simulink model "lab2_1"  (R2020b)
settings: Solver=VariableStepAuto  StartTime=0.0  StopTime=10.0  RelTol=1e-3
values from neighbouring files (symbols this model uses):
  g = 9.81    [lab2.m]
  km = 0.1    [lab2.m]
  La = 0.05    [lab2.m]
  M = 0.1    [lab2.m]
  Ra = 3    [lab2.m]
settings Model: Creator=shineofanuglyjewel  LastModifiedBy=shineofanuglyjewel
settings DebuggingCC: SFMachineParentedDataDiag=error

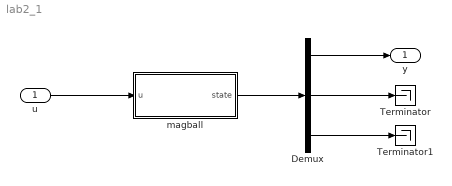
== system lab2_1 ==
  u : Inport  PortDimensions=1
  Demux : Demux  Outputs=3
  Terminator : Terminator
  Terminator1 : Terminator
  magball : Subsystem
  y : Outport
  wires:
  u/1 -> magball/1(u)
  Demux/1 -> y/1
  Demux/2 -> Terminator/1
  Demux/3 -> Terminator1/1
  magball/1(state) -> Demux/1

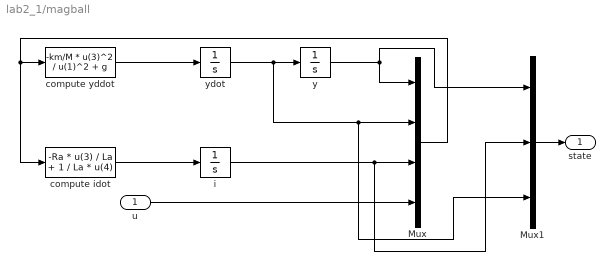
== system lab2_1/magball ==
  u : Inport
  Mux : Mux
  Mux1 : Mux  Inputs=3
  compute idot : MATLABFcn  MATLABFcn=-Ra * u(3) / La + 1 / La * u(4)
  compute yddot : MATLABFcn  MATLABFcn=-km/M * u(3)^2 / u(1)^2 + g
  i : Integrator
  y : Integrator
  ydot : Integrator
  state : Outport
  wires:
  compute yddot/1 -> ydot/1
  ydot/1 -> Mux1/3, Mux/2, y/1
  compute idot/1 -> i/1
  y/1 -> Mux1/1, Mux/1
  Mux1/1 -> state/1
  Mux/1 -> compute idot/1, compute yddot/1
  i/1 -> Mux/3, Mux1/2
  u/1 -> Mux/4
